simulink model "sldemo_solvers"  (Simulink 10.0)
settings: Solver=ode23s  StartTime=0.0  StopTime=86400  RelTol=1e-6  EnableMultiTasking=on
model workspace (MATLAB code in the model file):
  | g = 9.83;          % acceleration of gravity (m/sec^2)
  | L = 67;            % pendulum length (m)
  | initial_x = L/100; % initial x coordinate (m)
  | initial_y = 0;     % initial y coordinate (m)
  | initial_xdot = 0;  % initial x velocity (m/sec)
  | initial_ydot = 0;  % initial y velocity (m/sec)
  | Omega=2*pi/86400;  % Earth's angular velocity of rotation about its axis (rad/sec)
  | lambda=49/180*pi;  % latitude in (rad)
  | TotalEnergy = 1/2*(initial_xdot^2 + initial_ydot^2) + g*(L-sqrt( L^2-initial_x^2-initial_y^2)); % Calculate Total Energy
settings Model: Creator=The MathWorks, Inc.  LastModifiedBy=bhisma
settings SolverCC: SolverJacobianMethodControl=FullPerturbation
settings DataIOCC: SaveFormat=StructureWithTime  SaveOutput=off  SignalLogging=off  SaveTime=off  ReturnWorkspaceOutputs=on  SignalLoggingName=sldemo_slvers_output
settings OptimizationCC: ExpressionDepthLimit=2147483647  InitFltsAndDblsToZero=on
settings DebuggingCC: SaveWithParameterizedLinksMsg=none  SignalResolutionControl=TryResolveAllWithWarning  FcnCallInpInsideContextMsg=warning  StateNameClashWarn=warning  PregeneratedLibrarySubsystemCodeDiagnostic=none
settings HardwareCC: TargetBitPerLong=64  TargetBitPerPointer=64  TargetBitPerSizeT=64  TargetBitPerPtrDiffT=64  TargetLongLongMode=on  TargetIntDivRoundTo=Zero  TargetEndianess=LittleEndian  TargetWordSize=64  TargetHWDeviceType=MATLAB Host  ProdEqTarget=off
settings RTWCC: Description=Rapid Simulation Target  SystemTargetFile=rsim.tlc  TemplateMakefile=rsim_default_tmf
settings RSimTargetCC: TargetFcnLib=ansi_tfl_tmw.mat  PreserveStateflowLocalDataDimensions=off  RSIM_SOLVER_SELECTION=UseSolverModule
settings ConfigComp: CovExternalEMLEnable=off  CovSFcnEnable=off

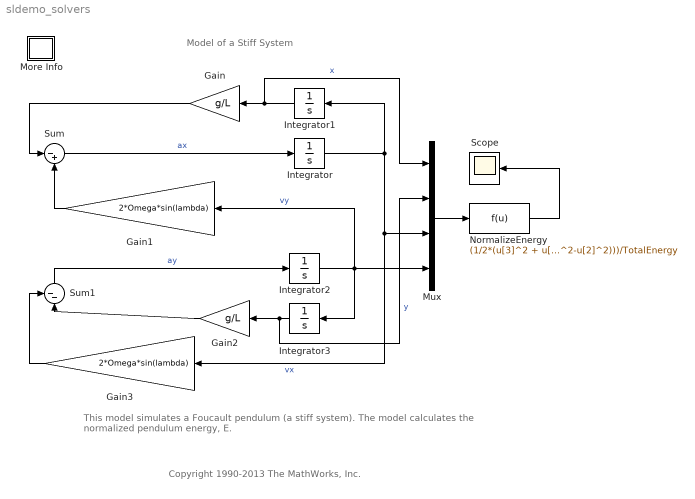
== system sldemo_solvers ==
  note: This model simulates a Foucault pendulum (a stiff system).
      | The model calculates the normalized pendulum energy, E.
  note: Model of a Stiff System
  note: Copyright 1990-2013 The MathWorks, Inc.
  Gain : Gain  Gain=g/L
  Gain1 : Gain  Gain=2*Omega*sin(lambda)
  Gain2 : Gain  Gain=g/L
  Gain3 : Gain  Gain=2*Omega*sin(lambda)
  Integrator : Integrator  InitialCondition=initial_xdot
  Integrator1 : Integrator  InitialCondition=initial_x
  Integrator2 : Integrator  InitialCondition=initial_ydot
  Integrator3 : Integrator  InitialCondition=initial_y
  More Info : Subsystem
      settings: OpenFcn=showExample('simulink_general/sldemo_solversExample')
      mask Display: disp('?')
  Mux : Mux
  NormalizeEnergy : Fcn  Expr=(1/2*(u[3]^2 + u[4]^2) + g*(L-sqrt( L^2-u[1]^2-u[2]^2)))/TotalEnergy
  Scope : Scope
  Sum : Sum  Inputs=|-+
  Sum1 : Sum  Inputs=--|
  wires:
  Integrator/1 -> Integrator1/1, Gain3/1, Mux/3  "vx"
  Integrator1/1 -> Gain/1, Mux/1  "x"
  Sum/1 -> Integrator/1  "ax"
  Gain/1 -> Sum/1
  Gain1/1 -> Sum/2
  Integrator2/1 -> Integrator3/1, Mux/4, Gain1/1  "vy"
  Gain2/1 -> Sum1/2
  Gain3/1 -> Sum1/1
  Sum1/1 -> Integrator2/1  "ay"
  Integrator3/1 -> Gain2/1, Mux/2  "y"
  Mux/1 -> NormalizeEnergy/1
  NormalizeEnergy/1 -> Scope/1

== system sldemo_solvers/More Info ==
